simulink subsystem "Truth"  (R2024b)
settings: Solver=VariableStepAuto  StartTime=0.0  StopTime=10.0  RelTol=1e-3
libraries: sim3dlib x2
settings Model: Creator=Tong  LastModifiedBy=Tong

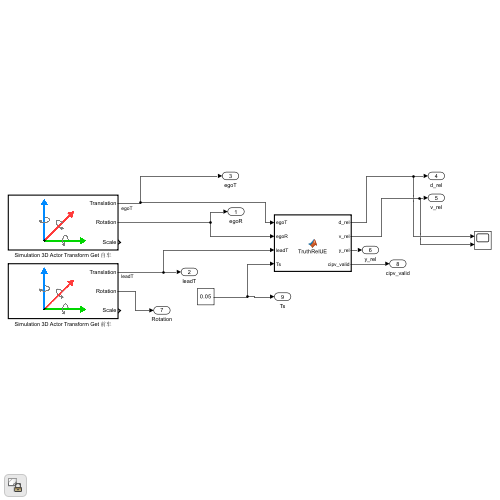
[thumbnail: Simulink's stored preview of the top-level diagram]
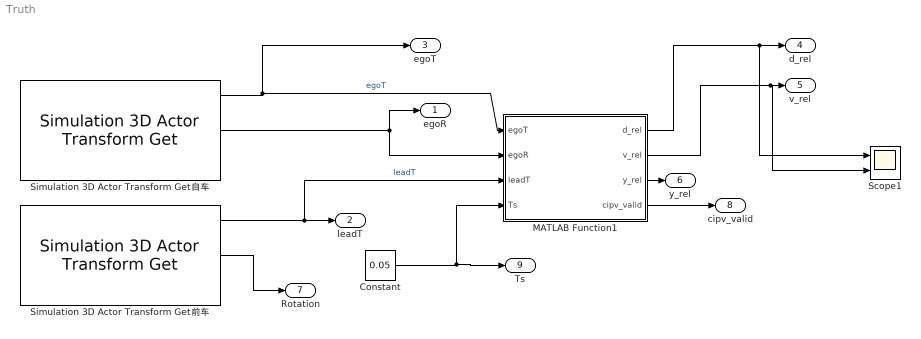
== system Truth ==
  Constant : Constant  Value=0.05
  MATLAB Function1 : MATLAB Function  TreatAsAtomicUnit=on
  Scope1 : Scope  NumInputPorts=2
  Simulation 3D Actor Transform Get 前车 : sim3dlib/Simulation 3D Actor Transform Get  Priority=1  ActorTag=SimulinkVehicle2  NumberOfParts=1  CustNumOfParts=3  Ts=0.05  aMode=5
      settings: LibrarySourceBlock=sl3dlib/Simulation 3D/Utilities/Simulation 3D Actor Transform Get
  Simulation 3D Actor Transform Get 自车 : sim3dlib/Simulation 3D Actor Transform Get  Priority=1  ActorTag=SimulinkVehicle1  NumberOfParts=1  CustNumOfParts=3  Ts=0.05  aMode=5
      settings: LibrarySourceBlock=sl3dlib/Simulation 3D/Utilities/Simulation 3D Actor Transform Get
  egoR : Outport
  leadT : Outport  Port=2
  egoT : Outport  Port=3
  d_rel : Outport  Port=4
  v_rel : Outport  Port=5
  y_rel : Outport  Port=6
  Rotation : Outport  Port=7
  cipv_valid : Outport  Port=8
  Ts : Outport  Port=9
  wires:
  MATLAB Function1/1(d_rel) -> d_rel/1, Scope1/1
  Simulation 3D Actor Transform Get 自车/2 -> MATLAB Function1/2(egoR), egoR/1
  Simulation 3D Actor Transform Get 前车/2 -> Rotation/1
  MATLAB Function1/4(cipv_valid) -> cipv_valid/1
  Simulation 3D Actor Transform Get 前车/1 -> leadT/1, MATLAB Function1/3(leadT)  "leadT"
  MATLAB Function1/2(v_rel) -> v_rel/1, Scope1/2
  Simulation 3D Actor Transform Get 自车/1 -> egoT/1, MATLAB Function1/1(egoT)  "egoT"
  MATLAB Function1/3(y_rel) -> y_rel/1
  Constant/1 -> MATLAB Function1/4(Ts), Ts/1

== matlab function Truth/MATLAB Function1 ==
  settings: updateMethod=DISCRETE
  data: egoT input; egoR input; leadT input; d_rel output; v_rel output; Ts input; y_rel output; cipv_valid output


% function [d_rel, v_rel, y_rel] = TruthRel(egoT, egoR, leadT, Ts)
% % egoT/leadT: [x y z] in world (m)
% % egoR: [roll pitch yaw] deg  OR quaternion [w x y z]
% persistent dPrev vFilt dFilt
% if isempty(dPrev)
%     dPrev = 0; vFilt = 0; dFilt = 0;
% end
% 
% % --- yaw from egoR ---
% yaw = 0;
% if numel(egoR)==3
%     yaw = deg2rad(egoR(3));
% elseif numel(egoR)==4
%     eul = quat2eul(egoR(:)');
%     yaw = eul(1);
% end
% 
% dp = leadT(1:2) - egoT(1:2);   % world delta in XY
% 
% % project world delta into ego forward/left
% dLong =  cos(yaw)*dp(1) + sin(yaw)*dp(2);   % forward distance
% dLat  = -sin(yaw)*dp(1) + cos(yaw)*dp(2);   % left positive
% 
% % low-pass on distance (2 Hz)
% alpha = exp(-2*pi*2*Ts);
% dFilt = alpha*dFilt + (1-alpha)*dLong;
% 
% % relative speed from derivative + low-pass
% vRaw  = (dFilt - dPrev)/Ts;
% dPrev = dFilt;
% 
% beta  = exp(-2*pi*2*Ts);
% vFilt = beta*vFilt + (1-beta)*vRaw;
% 
% % ================= 新增逻辑 =================
% % 车道过滤：只有在本车道（横向偏差 < 2米）才认为是前车
% Lane_Threshold = 2.0; 
% 
% if abs(dLat) < Lane_Threshold
%     % 目标在车道内，输出真实距离
%     d_rel = dFilt;
%     v_rel = vFilt;
% else
%     % 目标在车道外（隔壁车道），视为无前车
%     % 输出一个很大的距离，ACC 就会转为定速巡航，不受影响
%     d_rel = 200; 
%     v_rel = 0;
% end
% % ============================================
% 
% y_rel = dLat;



% function [d_rel, v_rel, y_rel, cipv_valid] = TruthRel(egoT, leadT, Xdot, Ydot, Ts)
% %#codegen
% % egoT/leadT: [x y z] world (m) —— 两者必须来自同一坐标系
% % Xdot,Ydot: ego 在同一坐标系下的速度分量 (m/s)
% % 输出:
% %   d_rel: 车前方纵向距离(沿车头方向投影)
% %   v_rel: 相对速度(对 d_rel 求导 + 滤波)
% %   y_rel: 横向偏差(左正)
% %   cipv_valid: 是否认为该车是前车
% 
% persistent dPrev vFilt dFilt isInit
% if isempty(isInit)
%     dPrev = 0; vFilt = 0; dFilt = 0; isInit = false;
% end
% 
% % 1) 用速度方向计算航向角（rad），避免 Rotation 坐标定义坑
% yaw = atan2(Ydot, Xdot);  % rad
% 
% % 2) 相对位移（世界坐标）
% dp = leadT(1:2) - egoT(1:2);
% 
% % 3) 投影到车体前向/左向
% dLong =  cos(yaw)*dp(1) + sin(yaw)*dp(2);   % forward
% dLat  = -sin(yaw)*dp(1) + cos(yaw)*dp(2);   % left+
% 
% % 4) 前车有效性：必须在前方且横向偏差在阈值内
% Lane_Threshold = 2.0; % m，可按车道宽稍调(1.8~2.5)
% cipv_valid = (dLong > 0) && (abs(dLat) < Lane_Threshold);
% 
% % 5) 初始化（第一次有效时把滤波器状态对齐，避免启动尖峰）
% if (~isInit) && cipv_valid
%     dFilt = dLong;
%     dPrev = dLong;
%     vFilt = 0;
%     isInit = true;
% end
% 
% % 6) 输出与滤波更新
% if cipv_valid && isInit
%     % 低通距离
%     alpha = exp(-2*pi*2*Ts);    % 2 Hz
%     dFilt = alpha*dFilt + (1-alpha)*dLong;
% 
%     % 由距离导数得到相对速度 + 低通
%     vRaw  = (dFilt - dPrev)/Ts;
%     dPrev = dFilt;
% 
%     beta  = exp(-2*pi*2*Ts);    % 2 Hz
%     vFilt = beta*vFilt + (1-beta)*vRaw;
% 
%     d_rel = dFilt;
%     v_rel = vFilt;
% else
%     % 无前车：给大距离，让 ACC 进入巡航；同时冻结/重置滤波，避免恢复时尖峰
%     d_rel = 1e6;
%     v_rel = 0;
%     vFilt = 0;
%     % dPrev/dFilt 不强行更新（冻结）
% end
% 
% y_rel = dLat;
% end


% function [d_rel, v_rel, y_rel, cipv_valid] = TruthRelUE(egoT, leadT, Ts)
% %#codegen
% % egoT/leadT: [x y z] from Simulation 3D Actor Transform Get (same UE frame)
% 
% persistent egoPrev leadPrev vFilt dFilt inited
% if isempty(inited)
%     egoPrev = egoT(1:2);
%     leadPrev = leadT(1:2);
%     vFilt = 0;
%     dFilt = 0;
%     inited = true;
% end
% 
% % 1) 由位置差分得到速度（UE 坐标系）
% egoV = (egoT(1:2) - egoPrev) / Ts;
% leadV = (leadT(1:2) - leadPrev) / Ts;
% egoPrev = egoT(1:2);
% leadPrev = leadT(1:2);
% 
% % 2) 航向角用 ego 速度方向（低速保持，防止乱跳）
% v = hypot(egoV(1), egoV(2));
% persistent yaw_last
% if isempty(yaw_last), yaw_last = 0; end
% 
% if v < 0.2
%     yaw = yaw_last;
% else
%     yaw = atan2(egoV(2), egoV(1)); % rad
%     yaw_last = yaw;
% end
% 
% % 3) 相对位移
% dp = leadT(1:2) - egoT(1:2);
% 
% % 4) 投影到 ego 前向/左向
% c = cos(yaw); s = sin(yaw);
% dLong =  c*dp(1) + s*dp(2);
% dLat  = -s*dp(1) + c*dp(2);
% 
% % 5) 有效性（前方 + 车道阈值）
% Lane_Threshold = 2.0;
% cipv_valid = (dLong > 0) && (abs(dLat) < Lane_Threshold);
% 
% % 6) 相对速度：投影相对速度向量（更稳）
% vRelRaw = c*(leadV(1)-egoV(1)) + s*(leadV(2)-egoV(2));
% 
% % 7) 低通（可选）
% alpha = exp(-2*pi*2*Ts);
% dFilt = alpha*dFilt + (1-alpha)*dLong;
% 
% beta = exp(-2*pi*2*Ts);
% vFilt = beta*vFilt + (1-beta)*vRelRaw;
% 
% if cipv_valid
%     d_rel = dFilt;
%     v_rel = vFilt;
% else
%     d_rel = 1e6;
%     v_rel = 0;
%     vFilt = 0;
% end
% 
% y_rel = dLat;
% end



% function [d_rel, v_rel, y_rel, cipv_valid] = TruthRelUE(egoT, leadT, Ts)
% %#codegen
% 
% persistent egoPrev leadPrev vFilt dFilt inited yaw_last
% if isempty(inited)
%     egoPrev = egoT(1:2);
%     leadPrev = leadT(1:2);
%     vFilt = 0;
%     dFilt = 0;
%     yaw_last = 0;
%     inited = true;
% end
% 
% % 1) 位置差分得到速度（UE）
% egoV = (egoT(1:2) - egoPrev) / Ts;
% leadV = (leadT(1:2) - leadPrev) / Ts;
% egoPrev = egoT(1:2);
% leadPrev = leadT(1:2);
% 
% % 2) 航向角：速度方向（低速保持）
% v = hypot(egoV(1), egoV(2));
% if v >= 0.2
%     yaw_last = atan2(egoV(2), egoV(1)); % rad
% end
% yaw = yaw_last;
% 
% % 3) 相对位移
% dp = leadT(1:2) - egoT(1:2);
% 
% % 4) 投影
% c = cos(yaw); s = sin(yaw);
% dLong =  c*dp(1) + s*dp(2);
% dLat  = -s*dp(1) + c*dp(2);
% 
% % 5) 有效性
% Lane_Threshold = 2.0;
% cipv_valid = (dLong > 0) && (abs(dLat) < Lane_Threshold);
% 
% % 6) 相对速度：投影相对速度向量
% vRelRaw = c*(leadV(1)-egoV(1)) + s*(leadV(2)-egoV(2));
% 
% % 7) 只在 valid 时滤波 & 输出；invalid 时输出巡航并冻结/重置
% alpha = exp(-2*pi*2*Ts);
% beta  = exp(-2*pi*2*Ts);
% 
% if cipv_valid
%     % 首次进入 valid：对齐初值，避免从0滤上去导致误刹
%     if dFilt == 0
%         dFilt = dLong;
%         vFilt = vRelRaw;
%     else
%         dFilt = alpha*dFilt + (1-alpha)*dLong;
%         vFilt = beta*vFilt + (1-beta)*vRelRaw;
%     end
% 
%     d_rel = dFilt;
%     v_rel = vFilt;
% else
%     d_rel = 1e6;   % 无前车 -> 巡航
%     v_rel = 0;
% 
%     % 关键：建议冻结或轻微重置，避免下一次 valid 输出污染值
%     % vFilt = 0;   % 可选：重置相对速度滤波
%     % dFilt = 0;   % 可选：重置距离滤波（更激进）
% end
% 
% y_rel = dLat;
% end


% function [d_rel, v_rel, y_rel, cipv_valid] = TruthRelUE_Fixed(egoT, egoR, leadT, Ts)
% %#codegen
% % UE真值：gap距离 + 低速yaw兜底 + valid防抖 + invalid不更新状态
% 
% % 车辆长度（按你actor长度改，Sedan常用4.7）
% Lego  = 4.7;
% Llead = 4.7;
% bumperComp = 0.5*Lego + 0.5*Llead;  % 中心距->保险杠距补偿
% 
% persistent egoPrev leadPrev yaw_last dFilt vFilt validCnt init
% if isempty(init)
%     egoPrev = egoT(1:2);
%     leadPrev = leadT(1:2);
%     yaw_last = deg2rad(egoR(3));  % 用Rotation初始化
%     dFilt = 0; vFilt = 0;
%     validCnt = 0;
%     init = true;
% end
% 
% % 1) UE速度（差分）
% egoV  = (egoT(1:2)  - egoPrev)  / Ts;
% leadV = (leadT(1:2) - leadPrev) / Ts;
% egoPrev  = egoT(1:2);
% leadPrev = leadT(1:2);
% 
% v = hypot(egoV(1), egoV(2));
% 
% % 2) 航向角：高速用速度方向，低速用Rotation yaw
% yawR = deg2rad(egoR(3));
% if v >= 0.5
%     yaw_last = atan2(egoV(2), egoV(1));
% else
%     yaw_last = yawR;
% end
% yaw = yaw_last;
% 
% % 3) 相对位移
% dp = leadT(1:2) - egoT(1:2);
% 
% % 4) 投影（中心距）
% c = cos(yaw); s = sin(yaw);
% dLong_center =  c*dp(1) + s*dp(2);
% dLat         = -s*dp(1) + c*dp(2);
% 
% % 5) gap（保险杠到保险杠）
% dLong_gap = dLong_center - bumperComp;
% 
% % 6) valid：前方 + 车道阈值 + 距离上限
% LaneTh = 2.0;
% dMax   = 200;
% validNow = (dLong_gap > 0) && (dLong_gap < dMax) && (abs(dLat) < LaneTh);
% 
% % 防抖：连续N帧valid才置真
% Nhold = 3;
% if validNow
%     validCnt = min(validCnt+1, Nhold);
% else
%     validCnt = 0;
% end
% cipv_valid = (validCnt >= Nhold);
% 
% % 7) 相对速度（投影相对速度向量）
% vRelRaw = c*(leadV(1)-egoV(1)) + s*(leadV(2)-egoV(2));
% 
% % 8) 只在valid时更新滤波；invalid时重置（防鬼刹）
% alpha = exp(-2*pi*2*Ts);
% beta  = exp(-2*pi*2*Ts);
% 
% if cipv_valid
%     if dFilt == 0
%         dFilt = dLong_gap;
%         vFilt = vRelRaw;
%     else
%         dFilt = alpha*dFilt + (1-alpha)*dLong_gap;
%         vFilt = beta*vFilt + (1-beta)*vRelRaw;
%     end
%     d_rel = dFilt;
%     v_rel = vFilt;
% else
%     d_rel = 1e6;
%     v_rel = 0;
%     dFilt = 0;
%     vFilt = 0;
% end
% 
% y_rel = dLat;
% end



% function [d_rel, v_rel, y_rel, cipv_valid] = TruthRelUE_Fixed(egoT, egoR, leadT, Ts)
% %#codegen
% 
% Lego  = 4.7;
% Llead = 4.7;
% bumperComp = 0.5*Lego + 0.5*Llead;
% 
% persistent egoPrev leadPrev yaw_last dFilt vFilt init
% persistent validState cntOn cntOff
% 
% if isempty(init)
%     egoPrev = egoT(1:2);
%     leadPrev = leadT(1:2);
%     yaw_last = deg2rad(egoR(3));
%     dFilt = 0; vFilt = 0;
%     validState = false;
%     cntOn = 0; cntOff = 0;
%     init = true;
% end
% 
% % --- 速度（UE差分）---
% egoV  = (egoT(1:2)  - egoPrev)  / Ts;
% leadV = (leadT(1:2) - leadPrev) / Ts;
% egoPrev  = egoT(1:2);
% leadPrev = leadT(1:2);
% 
% v = hypot(egoV(1), egoV(2));
% 
% % --- yaw：高速用速度方向，低速用Rotation兜底 ---
% yawR = deg2rad(egoR(3));
% if v >= 0.5
%     yaw_last = atan2(egoV(2), egoV(1));
% else
%     % yaw_last = yawR;
% end
% yaw = yaw_last;
% 
% % --- 相对位移与投影 ---
% dp = leadT(1:2) - egoT(1:2);
% c = cos(yaw); s = sin(yaw);
% dLong_center =  c*dp(1) + s*dp(2);
% dLat         = -s*dp(1) + c*dp(2);
% 
% % gap
% dLong = dLong_center - bumperComp;
% 
% % ===================== 关键：valid 滞回 + 防抖锁存 =====================
% % 进入阈值要“更严格”，退出阈值更“宽松”
% LaneEnter = 1.8;   % 进入车道判定阈值（小）
% LaneExit  = 2.3;   % 退出阈值（大）
% dMaxEnter = 180;
% dMaxExit  = 220;
% 
% % on/off 防抖帧数（Ts=0.05，3帧=0.15s）
% Non  = 3;
% Noff = 10;
% 
% if validState
%     validNow = (dLong > 0) && (dLong < dMaxExit) && (abs(dLat) < LaneExit);
% else
%     validNow = (dLong > 0) && (dLong < dMaxEnter) && (abs(dLat) < LaneEnter);
% end
% 
% if validNow
%     cntOn  = min(cntOn+1, Non);
%     cntOff = 0;
% else
%     cntOff = min(cntOff+1, Noff);
%     cntOn  = 0;
% end
% 
% if ~validState && (cntOn >= Non)
%     validState = true;
% elseif validState && (cntOff >= Noff)
%     validState = false;
% end
% 
% cipv_valid = validState;
% % ======================================================================
% 
% % --- 相对速度（投影相对速度向量）---
% vRelRaw = c*(leadV(1)-egoV(1)) + s*(leadV(2)-egoV(2));
% 
% % --- 滤波（只在 valid 时更新；invalid 重置）---
% alpha = exp(-2*pi*2*Ts);
% beta  = exp(-2*pi*2*Ts);
% 
% if cipv_valid
%     if dFilt == 0
%         dFilt = dLong;
%         vFilt = vRelRaw;
%     else
%         dFilt = alpha*dFilt + (1-alpha)*dLong;
%         vFilt = beta*vFilt + (1-beta)*vRelRaw;
%     end
%     d_rel = dFilt;
%     v_rel = vFilt;
% else
%     d_rel = 200;
%     v_rel = 0;
%     dFilt = 0;
%     vFilt = 0;
% end
% 
% y_rel = dLat;
% end




% function [d_rel, v_rel, y_rel, cipv_valid] = TruthRelUE_Fixed(egoT, egoR, leadT, Ts)
% %#codegen
% % egoT/leadT: [x y z] from Simulation 3D Actor Transform Get (same frame)
% % egoR: [roll pitch yaw] in degrees (UE rotation) - 本版本不再使用 egoR
% % 输出 d_rel 为 gap(保险杠距)
% 
% %% ---------- 参数区 ----------
% Lego  = 4.7;
% Llead = 4.7;
% bumperComp = 0.5*Lego + 0.5*Llead;   % center distance -> bumper-to-bumper gap
% 
% % 车道判定滞回
% LaneEnter = 1.8;
% LaneExit  = 2.3;
% dMaxEnter = 180;
% dMaxExit  = 220;
% 
% % valid 防抖
% Non  = 3;
% Noff = 10;
% 
% % 速度差分滤波（关键：压 v_rel 台阶）
% fcV = 5;                 % Hz，速度滤波截止频率(3~8Hz可调)
% alphaV = exp(-2*pi*fcV*Ts);
% 
% % 距离/相对速度输出滤波
% fcOut = 2;               % Hz(1~3Hz可调)
% alphaD = exp(-2*pi*fcOut*Ts);
% alphaVr = exp(-2*pi*fcOut*Ts);
% 
% % yaw 纯速度方向计算参数
% vHoldYaw   = 0.5;         % m/s 低于此速度保持上一次航向
% maxYawRate = deg2rad(120);% rad/s，yaw变化率限幅
% alphaYaw   = 0.85;        % 航向滤波系数(0~1，越大越平滑)
% 
% % invalid 输出策略
% NO_TARGET_DIST = 200;     
% %% ----------------------------
% 
% %% ---------- 持久变量 ----------
% persistent egoPrev leadPrev egoVf leadVf yawF dFilt vFilt init yawInit
% persistent validState cntOn cntOff lostCnt
% 
% if isempty(init)
%     egoPrev = egoT(1:2)';   
%     leadPrev = leadT(1:2)'; 
%     egoVf = [0;0];
%     leadVf = [0;0];
% 
%     yawF = 0;               % 初始航向设为0
%     yawInit = false;        % 未曾获得有效航向
% 
%     dFilt = 0;
%     vFilt = 0;
% 
%     validState = false;
%     cntOn = int32(0);
%     cntOff = int32(0);
%     lostCnt = int32(0);
% 
%     init = true;
% end
% 
% %% ---------- 1) 速度估计 + 低通（抑制差分台阶） ----------
% egoVraw  = (egoT(1:2)'  - egoPrev)  / Ts;   
% leadVraw = (leadT(1:2)' - leadPrev) / Ts;   
% egoPrev  = egoT(1:2)';                       
% leadPrev = leadT(1:2)';                      
% 
% egoVf  = alphaV*egoVf  + (1-alphaV)*egoVraw;
% leadVf = alphaV*leadVf + (1-alphaV)*leadVraw;
% 
% vEgo = hypot(egoVf(1), egoVf(2));
% 
% %% ---------- 2) yaw：纯速度方向 + 低速保持 + 限幅 + 滤波 ----------
% if vEgo >= vHoldYaw
%     % 高速：计算速度方向
%     yawMeas = atan2(egoVf(2), egoVf(1));
% 
%     % 首次有效速度：直接赋值，防止从0跳变
%     if ~yawInit
%         yawF = yawMeas;
%         yawInit = true;
%     end
% else
%     % 低速：保持上一次航向
%     yawMeas = yawF;
% end
% 
% % 只在有效速度时进行滤波和限幅更新
% if yawInit && vEgo >= vHoldYaw
%     % 角度差（考虑wrap）
%     eYaw = wrapToPi(yawMeas - yawF);
% 
%     % 角速度限幅（防瞬跳）
%     maxStep = maxYawRate * Ts;
%     if eYaw >  maxStep, eYaw =  maxStep; end
%     if eYaw < -maxStep, eYaw = -maxStep; end
% 
%     % 一阶滤波（在受限误差上滤）
%     yawF = wrapToPi(yawF + (1-alphaYaw)*eYaw);
% end
% 
% c = cos(yawF); s = sin(yawF);
% 
% %% ---------- 3) 相对位移投影 + gap ----------
% dp = leadT(1:2)' - egoT(1:2)';   
% dLong_center =  c*dp(1) + s*dp(2);
% dLat         = -s*dp(1) + c*dp(2);
% 
% dLong_gap = dLong_center - bumperComp;
% if dLong_gap < 0
%     dLong_gap = 0;  
% end
% 
% %% ---------- 4) valid 滞回 + 防抖 ----------
% if validState
%     validNow = (dLong_gap > 0) && (dLong_gap < dMaxExit)  && (abs(dLat) < LaneExit);
% else
%     validNow = (dLong_gap > 0) && (dLong_gap < dMaxEnter) && (abs(dLat) < LaneEnter);
% end
% 
% if validNow
%     cntOn  = min(cntOn+1, int32(Non));
%     cntOff = int32(0);
% else
%     cntOff = min(cntOff+1, int32(Noff));
%     cntOn  = int32(0);
% end
% 
% if (~validState) && (cntOn >= Non)
%     validState = true;
% elseif validState && (cntOff >= Noff)
%     validState = false;
% end
% cipv_valid = validState;
% 
% %% ---------- 5) 相对速度：投影相对速度向量 + 滤波 ----------
% vRelRaw = c*(leadVf(1)-egoVf(1)) + s*(leadVf(2)-egoVf(2));
% 
% if cipv_valid
%     lostCnt = int32(0);
% 
%     if dFilt == 0
%         dFilt = dLong_gap;
%         vFilt = vRelRaw;
%     else
%         dFilt = alphaD*dFilt + (1-alphaD)*dLong_gap;
%         vFilt = alphaVr*vFilt + (1-alphaVr)*vRelRaw;
%     end
% 
%     d_rel = dFilt;
%     v_rel = vFilt;
% 
% else
%     N_keep = int32(round(0.3 / Ts));
%     if lostCnt < N_keep && dFilt > 0
%         lostCnt = lostCnt + 1;
%         d_rel = dFilt;
%         v_rel = vFilt;
%     else
%         d_rel = NO_TARGET_DIST;
%         v_rel = 0;
%         dFilt = 0;
%         vFilt = 0;
%         lostCnt = int32(0);
%     end
% end
% 
% y_rel = dLat;
% 
% end
% 
% %% ---------- helper ----------
% function y = wrapToPi(x)
% y = mod(x+pi, 2*pi) - pi;
% end



function [d_rel, v_rel, y_rel, cipv_valid] = TruthRelUE(egoT, egoR, leadT, Ts)
%#codegen
% TruthRelUE_Fixed
% 基于UE Actor Transform计算前车相对状态（控制友好输出）
% 输出:
%   d_rel      - 前车gap距离(保险杠到保险杠, m)，无目标时置NO_TARGET_DIST
%   v_rel      - 相对速度(lead-ego, m/s)，无目标时置0
%   y_rel      - 横向偏差(左正, m)
%   cipv_valid - 目标有效标志（含滞回+防抖）
%
% 说明：
% 1) 保持原功能逻辑不变；
% 2) 车道限制/滞回逻辑仅用于控制输出稳定性；
% 3) 代码结构优化，便于后续参数标定与维护。

%% ================= 参数区 =================
% 车辆几何（中心距 -> 保险杠间隙补偿）
Lego  = 4.7;
Llead = 4.7;
bumperComp = 0.5 * (Lego + Llead);

% 车道判定滞回
LaneEnter = 1.8;
LaneExit  = 2.3;
dMaxEnter = 180;
dMaxExit  = 220;

% 有效性防抖
Non  = int32(3);   % 连续Non帧满足进入
Noff = int32(10);  % 连续Noff帧不满足退出

% 速度差分滤波（抑制台阶）
fcV = 5; % Hz
alphaV = exp(-2*pi*fcV*Ts);

% 输出滤波
fcOut = 2; % Hz
alphaD  = exp(-2*pi*fcOut*Ts);
alphaVr = exp(-2*pi*fcOut*Ts);

% 航向估计
vHoldYaw   = 0.5;            % m/s 低于该速度保持航向
maxYawRate = deg2rad(120);   % rad/s 航向变化率限幅
alphaYaw   = 0.85;           % 航向一阶滤波系数

% 无目标控制占位
NO_TARGET_DIST = 200;

% 丢目标短时保持
N_keep = int32(round(0.3 / Ts));
%% =========================================

%% ================= 持久变量 =================
persistent init
persistent egoPrev leadPrev          % 上一帧位置(2x1)
persistent egoVf leadVf              % 滤波后速度(2x1)
persistent yawF yawInit              % 航向状态
persistent dFilt vFilt               % 控制输出滤波状态
persistent validState cntOn cntOff   % valid滞回状态机
persistent lostCnt                   % 丢目标保持计数

if isempty(init)
    egoPrev = egoT(1:2)';
    leadPrev = leadT(1:2)';

    egoVf = [0; 0];
    leadVf = [0; 0];

    yawF = deg2rad(egoR(3)); % 用旋转角初始化
    yawInit = true;

    dFilt = 0;
    vFilt = 0;

    validState = false;
    cntOn = int32(0);
    cntOff = int32(0);

    lostCnt = int32(0);
    init = true;
end
%% ==========================================

%% 1) 速度估计 + 低通
egoNow  = egoT(1:2)';
leadNow = leadT(1:2)';

egoVraw  = (egoNow  - egoPrev)  / Ts;
leadVraw = (leadNow - leadPrev) / Ts;

egoPrev  = egoNow;
leadPrev = leadNow;

egoVf  = alphaV * egoVf  + (1 - alphaV) * egoVraw;
leadVf = alphaV * leadVf + (1 - alphaV) * leadVraw;

vEgo = hypot(egoVf(1), egoVf(2));

%% 2) 航向估计：速度方向 + 限幅 + 滤波
if vEgo >= vHoldYaw
    yawMeas = atan2(egoVf(2), egoVf(1));
    if ~yawInit
        yawF = yawMeas;
        yawInit = true;
    end
else
    yawMeas = yawF; % 低速保持
end

if yawInit && (vEgo >= vHoldYaw)
    eYaw = wrapToPiLocal(yawMeas - yawF);

    maxStep = maxYawRate * Ts;
    if eYaw >  maxStep, eYaw =  maxStep; end
    if eYaw < -maxStep, eYaw = -maxStep; end

    yawF = wrapToPiLocal(yawF + (1 - alphaYaw) * eYaw);
end

c = cos(yawF);
s = sin(yawF);

%% 3) 相对位移投影 + gap
dp = leadNow - egoNow; % world XY

dLong_center =  c * dp(1) + s * dp(2);
dLat         = -s * dp(1) + c * dp(2);

dLong_gap = dLong_center - bumperComp;
if dLong_gap < 0
    dLong_gap = 0;
end

%% 4) valid滞回 + 防抖
if validState
    validNow = (dLong_gap > 0) && (dLong_gap < dMaxExit)  && (abs(dLat) < LaneExit);
else
    validNow = (dLong_gap > 0) && (dLong_gap < dMaxEnter) && (abs(dLat) < LaneEnter);
end

if validNow
    cntOn  = min(cntOn + 1, Non);
    cntOff = int32(0);
else
    cntOff = min(cntOff + 1, Noff);
    cntOn  = int32(0);
end

if (~validState) && (cntOn >= Non)
    validState = true;
elseif validState && (cntOff >= Noff)
    validState = false;
end

cipv_valid = validState;

%% 5) 相对速度（投影相对速度向量）
vRelRaw = c * (leadVf(1) - egoVf(1)) + s * (leadVf(2) - egoVf(2));

%% 6) 控制输出（保持原策略）
if cipv_valid
    lostCnt = int32(0);

    if dFilt == 0
        % 首次有效对齐，避免滤波启动尖峰
        dFilt = dLong_gap;
        vFilt = vRelRaw;
    else
        dFilt = alphaD  * dFilt + (1 - alphaD)  * dLong_gap;
        vFilt = alphaVr * vFilt + (1 - alphaVr) * vRelRaw;
    end

    d_rel = dFilt;
    v_rel = vFilt;

else
    % 短时保持，避免控制抖动
    if (lostCnt < N_keep) && (dFilt > 0)
        lostCnt = lostCnt + 1;
        d_rel = dFilt;
        v_rel = vFilt;
    else
        d_rel = NO_TARGET_DIST;
        v_rel = 0;

        dFilt = 0;
        vFilt = 0;
        lostCnt = int32(0);
    end
end

y_rel = dLat;

end

%% ============== 本地工具函数 ==============
function y = wrapToPiLocal(x)
y = mod(x + pi, 2*pi) - pi;
end
